simulink model "Control_Jetson_10ms_21b 1"  (R2021b)
settings: Solver=ode4  StartTime=0.0  StopTime=10  FixedStep=0.01  MaxStep=0  RelTol=1e-5  AbsTol=1e-3
InitFcn:
  | % Carrega parâmetros gerais (Massa, Ganhos PID, Geometria)
  | run('Parameters.m');
  | 
  | % Carrega as Tabelas (Lookup Tables)
  | run('curva_steering.m');
  | run('curva_tq_motor.m');
  | Ts = 0.001;
  | % (Opcional) Mensagem no Command Window para confirmar que rodou
  | disp('--- Parâmetros e Curvas Carregados com Sucesso ---');
model workspace (MAT data in the model file):
  A = 1.22
  Ack = 1
  Cd = 1.1
  Cl = -2
  Cs = [19075.58 25992.8 31792.64 35898.02 39044.37]
  Fz0x = -811.9083
  Fz0y = -210.9467
  Fz_cs = [222.41 444.82 667.23 889.64 1112.05]
  IAY = 0
  IAx = 0
  IAy = 0
  Im = 0.00033
  It = 0.0094
  Iw = 0.1578
  Iw_ = 0.7
  Iz_car = 150
  K_50_understeer = 0.005184
  K_Stability = 1
  K_oversteer = -0.001
  Kappa_F = 0
  Kappa_R = 0
  Km_FM = 110000
  Km_Fm = 110000
  Km_RM = 120000
  Km_Rm = 120000
  KphiARB_F = 0
  KphiARB_R = 11000
  KphiF = 1068.14
  KphiR = 1637.12
  Kphim_F = 137500
  Kphim_R = 48600
  L = 1.53
  M = 300
  Mgt = 11.72
  Mz_maxF = [0 66.3 132.6 198.9 265.2 330.23 396.52 462.83 529.112 595.42 661.73 728.03 ... (26 elements, 1x26)]
  Mz_minF = [0 -66.3 -132.6 -198.9 -265.2 -330.23 -396.52 -462.83 -529.112 -595.42 -661.73 -728.03 ... (26 elements, 1x26)]
  P = 68.9476
  P0 = 55.4852
  R = 0.2032
  Rcurva = 20
  Re = 0.2
  SR = 3
  TV_On = 1
  Ts = 0.01
  W = 2940
  Wf = 661.5
  Wr = 808.5
  Ws = 2324
  YLL = 1.11022302463e-16
  cx1 = 1.3668
  cy1 = 1.839
  dpi = 0.242630467224
  dx1 = 2.1568
  dx2 = -0.065814
  dx3 = 0.0011254
  dy1 = 2.453
  dy2 = -0.11197
  dy3 = 10.2899
  ex1 = -0.19815
  ex2 = -0.62529
  ex3 = 1.3396
  ex4 = 0.0029464
  ey1 = 0.96085
  ey2 = -0.28662
  ey3 = 0.14389
  ey4 = 4.9274
  ey5 = -70.7165
  g = 9.8
  hcg = 0.28495
  hcgs = 0.202
  hrc_f = 0.065
  hrc_r = 0.094
  hs_f = 0.245
  hs_r = 0.21
  hx1 = -0.003859
  hx2 = -0.000374
  hy1 = -0.000403
  hy2 = -0.000261
  kx1 = -36.9039
  kx2 = 22.3857
  kx3 = 0.61844
  ky1 = -83.2526
  ky2 = -5.565
  ky3 = 0.88491
  ky4 = 2.9994
  ky5 = -99.9393
  ky6 = -3.4705
  ky7 = -0.91452
  lf = 0.8415
  lr = 0.6885
  mass_FL = 67.5
  mass_FR = 67.5
  mass_RL = 82.5
  mass_RR = 82.5
  mi = 2
  ms = 240
  pedal = [0 1 2 3 4 5 6 7 8 9 10 11 ... (26 elements, 1x26)]
  pty1 = 0.005744
  pty2 = 19.1334
  px1 = -0.039964
  px2 = -0.15015
  px3 = -0.32528
  px4 = -0.063273
  py1 = 0.38578
  py2 = 1.2048
  py3 = -0.14544
  py4 = 0.092886
  py5 = -0.82901
  r = 9
  rhoar = 1.22
  s_f = 1
  s_r = 0.9
  tf = 1.2
  tr = 1.18
  vx1 = -0.11922
  vx2 = 0.002205
  vy1 = 0.032907
  vy2 = 0.018068
  vy3 = -1.0429
  vy4 = 0.53712
  x_fl = 0.8415
  x_fr = 0.8415
  x_rl = 0.6885
  x_rr = 0.6885
  xs_f = 0.89
  xs_r = 0.638
  y_fl = 0.6
  y_fr = 0.6
  y_rl = 0.59
  y_rr = 0.59
undefined symbols (not defined in the file or in its folder): Gr, K_t, K_variavel, Ki_data, Kp_data, magnitude, rpm, torque, Vx, Vx_axis
libraries: simulink x10, fuzblock x4
(part 2 of 2)

== system Control_Jetson_10ms_21b 1/Controle/Traction Control/Subsystem/Velocity Margin3/dfz ==
  Constant : Constant  Value=Fz0x
  Divide : Product  Inputs=*/
  Gain : Gain  Gain=-1
  Sum : Sum  Inputs=|+-
  tag scope: dfz_rr=global
  wires:
  Sum/1 -> Divide/1
  Divide/1 -> [dfz_rr]
  Constant/1 -> Sum/2, Divide/2
  [Fz_RR] -> Gain/1
  Gain/1 -> Sum/1

== matlab function Control_Jetson_10ms_21b 1/Controle/Weight Transfer /MATLAB Function1 ==
  data: u input; y output
function y = fcn(u)
    if u < 0 
        u = 0;
    else 
        y = u;
    end
y = u;

== matlab function Control_Jetson_10ms_21b 1/Controle/Weight Transfer /MATLAB Function2 ==
  data: u input; y output
function y = fcn(u)
    if u < 0 
        u = 0;
    else 
        y = u;
    end
y = u;

== matlab function Control_Jetson_10ms_21b 1/Controle/Weight Transfer /MATLAB Function3 ==
  data: u input; y output
function y = fcn(u)
    if u < 0 
        u = 0;
    else 
        y = u;
    end
y = u;

== matlab function Control_Jetson_10ms_21b 1/Controle/Weight Transfer /MATLAB Function4 ==
  data: u input; y output
function y = fcn(u)

if u <= 0
    y = 0;
else
    y = u;
end

== matlab function Control_Jetson_10ms_21b 1/Controle/Weight Transfer /MATLAB Function5 ==
  data: u input; y output
function y = fcn(u)

if u <= 0
    y = 0;
else
    y = u;
end

== matlab function Control_Jetson_10ms_21b 1/Controle/Weight Transfer /MATLAB Function ==
  data: u input; y output
function y = fcn(u)
    if u < 0 
        u = 0;
    else 
        y = u;
    end
y = u;
